simulink model "Demo_CarRealTime2D_cs"  (R2014b)
settings: Solver=ode5  SolverMode=SingleTasking  StartTime=0.0  StopTime=inf  FixedStep=1/1000  RelTol=1e-3
PreLoadFcn:
  | mbxruntime.callbacks.PreLoadFcn(bdroot);
  | check_NUTS_defined;
  | assignin('base',['model_closed_' bdroot],false);
  | addpath('../includes_AEBS');
PostLoadFcn:
  | mbxruntime.callbacks.PostLoadFcn(bdroot);
InitFcn:
  | mbxruntime.callbacks.InitFcn(bdroot);
StartFcn:
  | mbxruntime.callbacks.StartFcn(bdroot);
StopFcn:
  | mbxruntime.callbacks.StopFcn(bdroot);;
  | 
model workspace: external: MAT-File .\Demo_CarRealTime2D_cs_hws.mat (data not in the file)
undefined symbols (not defined in the file or in its folder): Driver_Demands, mbxruntime, tabledata, vicrt_initcallback, vicrt_initmexcallback, vicrt_simulationmanager, warningInitialVelocity, x0
undefined symbols (not defined in the file): Demo_CarRealTime2D_cs_007c1c37f387f47f, Demo_CarRealTime2D_cs_085a64a83ba38cec, Demo_CarRealTime2D_cs_0a7f542d3fc7ab9f, Demo_CarRealTime2D_cs_0d7c72cfaa56dff7, Demo_CarRealTime2D_cs_0de07b35068e3828, Demo_CarRealTime2D_cs_17f4d381375cce95, Demo_CarRealTime2D_cs_1db40a09b08215a9, Demo_CarRealTime2D_cs_2bfa3850c176687b, Demo_CarRealTime2D_cs_35a34f1ba6ce4a22, Demo_CarRealTime2D_cs_378cc77e08d643fb, Demo_CarRealTime2D_cs_409b5c3befba0000, Demo_CarRealTime2D_cs_42628ca5bb62d2f3, Demo_CarRealTime2D_cs_56554a2db408a7f8, Demo_CarRealTime2D_cs_59527455249d7429, Demo_CarRealTime2D_cs_5983ee1b8112afac, Demo_CarRealTime2D_cs_5b5ebcf3ed7bf8e6, Demo_CarRealTime2D_cs_63cbe7fbe16cd5d9, Demo_CarRealTime2D_cs_6e17b9adbf989abf, Demo_CarRealTime2D_cs_6f662a34e5d9a196, Demo_CarRealTime2D_cs_75c4ee8892821e19, Demo_CarRealTime2D_cs_7c64486355814be2, Demo_CarRealTime2D_cs_849809550a2230ef, Demo_CarRealTime2D_cs_87f899bcbe16d8f5, Demo_CarRealTime2D_cs_8e7b50dac25b68a2, Demo_CarRealTime2D_cs_94938e5260f139b3, Demo_CarRealTime2D_cs_983acc940698d1d1, Demo_CarRealTime2D_cs_9d554c72797f76fd, Demo_CarRealTime2D_cs_9d747ee2f15c057f, Demo_CarRealTime2D_cs_ad62a2084d31e898, Demo_CarRealTime2D_cs_b56c8c5f000d30f0, Demo_CarRealTime2D_cs_b95f1b7356e926cc, Demo_CarRealTime2D_cs_BMW_X5_1_Path_pathUniqueID, Demo_CarRealTime2D_cs_BMW_Z3_2_Dynamics_Empty_STATE_BMW_Z3_2_x0, Demo_CarRealTime2D_cs_BMW_Z3_2_Dynamics_Empty_STATE_BMW_Z3_2_y0, Demo_CarRealTime2D_cs_BMW_Z3_2_Dynamics_Empty_STATE_BMW_Z3_2_z0, Demo_CarRealTime2D_cs_BMW_Z3_Path_pathUniqueID, Demo_CarRealTime2D_cs_BMW_Z3_SpeedProfile_speedProfileUniqueID, Demo_CarRealTime2D_cs_c8847ab2e5633224, Demo_CarRealTime2D_cs_c9a0d701286b93fb, Demo_CarRealTime2D_cs_ce758cae7dd1b283, Demo_CarRealTime2D_cs_CrossingPedestrian_Path_pathUniqueID, Demo_CarRealTime2D_cs_CuttingInVehicle_Path_pathUniqueID, Demo_CarRealTime2D_cs_d901ab1c1d2e40bc, Demo_CarRealTime2D_cs_dff70430e5a00a86, Demo_CarRealTime2D_cs_ef038a4f619ad32e, Demo_CarRealTime2D_cs_Female_OverweightAni_1_Path_pathUniqueID, Demo_CarRealTime2D_cs_Ford_Fiesta_1_Path_pathUniqueID, Demo_CarRealTime2D_cs_Ford_FocusWagon_Path_pathUniqueID, Demo_CarRealTime2D_cs_Sphere_1_Dynamics_Empty_STATE_Sphere_1_x0, Demo_CarRealTime2D_cs_Sphere_1_Dynamics_Empty_STATE_Sphere_1_y0, Demo_CarRealTime2D_cs_Sphere_1_Dynamics_Empty_STATE_Sphere_1_z0, WheelL0, WheelL1, WheelR0, WheelR1
libraries: PreScanSimulinkLibrary x15, simulink x15, simulink_extras x15, PreScanUsefulBlocks x2, dspsigops x1
(part 14 of 17)

== system Demo_CarRealTime2D_cs/HostVehicle/Dynamics_UserSpecified/VI-CarRealTime/Input_Bus/Bus2Map ==
  Bus In : Inport
  Bus Selector : BusSelector  OutputSignals=Driver_Demands.str_swa,Subsystem_Activation.Internal_Steering_Column_Activity,Driver_Demands.rack_displacement,Driver_Demands.throttle,Driver_Demands.gear,Driver_Demands.clutch,Driver_Demands.brake,Brake_System_General.brk_mast_cyl_pres,Brake_System_General.brk_bias_front,Driver_Demands.user_maneuver_ID,Driver_Demands.user_input_steering,Driver_Demands.user_input_throttle,Driver_Demands.user_input_braking,Driver_Demands.user_input_gear,Driver_Demands.user_input_clutch,Friction.tire_mu.L1,Friction.tire_mu.L2,Friction.tire_mu.R1,Friction.tire_mu.R2,Subsystem_Activation.Internal_Brake_System_Activity.L1,Brake_System.brk_mmag_sign.L1,Brake_System.brk_mmag_unsign.L1,Brake_System.brk_pres.L1,Brake_System.brk_pres_gain.L1,Brake_System.brk_mu.L1,Subsystem_Activation.Internal_Brake_System_Activity.L2,Brake_System.brk_mmag_sign.L2,Brake_System.brk_mmag_unsign.L2,Brake_System.brk_pres.L2,Brake_System.brk_pres_gain.L2,Brake_System.brk_mu.L2,Subsystem_Activation.Internal_Brake_System_Activity.R1,Brake_System.brk_mmag_sign.R1,Brake_System.brk_mmag_unsign.R1,Brake_System.brk_pres.R1,Brake_System.brk_pres_gain.R1,Brake_System.brk_mu.R1,Subsystem_Activation.Internal_Brake_System_Activity.R2,Brake_System.brk_mmag_sign.R2,Brake_System.brk_mmag_unsign.R2,Brake_System.brk_pres.R2,Brake_System.brk_pres_gain.R2,Brake_System.brk_mu.R2,Hook.Fx.rear,Hook.Fy.rear,Hook.Fz.rear,Hook.Mx.rear,Hook.My.rear,Hook.Mz.rear,Rear_Steering_Actuator_disp.str_swa.left,Rear_Steering_Actuator_disp.str_swa.right,Steering.steer_at_spindle.L1,Steering.steer_at_spindle.L2,Steering.steer_at_spindle.R1,Steering.steer_at_spindle.R2,Subsystem_Activation.Internal_Clutch_Activity,Subsystem_Activation.Internal_Engine_Activity,Subsystem_Activation.Internal_Gearbox_Activity,Engine.engine_omega,Engine.engine_max_trq,Engine.engine_min_trq,Engine.engine_trq,Engine.non_termic_engine_trq,GearBox.transmission_ratio,Clutch.clutch_trq,Clutch.clutch_slip_angle,Antiroll_Bar.activity_flag.front,Antiroll_Bar.activity_flag.rear,Antiroll_Bar.force.front,Antiroll_Bar.force.rear,Subsystem_Activation.Internal_Aero_Activity,Aerodynamic.fx_front,Aerodynamic.fy_front,Aerodynamic.fz_front,Aerodynamic.fx_rear,Aerodynamic.fy_rear,Aerodynamic.fz_rear,Aerodynamic.fx_center,Aerodynamic.fy_center,Aerodynamic.fz_center,Aerodynamic.mx,Aerodynamic.my,Aerodynamic.mz,Irregularity.road.L1,Irregularity.road.L2,Irregularity.road.R1,Irregularity.road.R2,Main_Damper.force.L1,Main_Damper.activity_flag.L1,Main_Damper.force.L2,Main_Damper.activity_flag.L2,Main_Damper.force.R1,Main_Damper.activity_flag.R1,Main_Damper.force.R2,Main_Damper.activity_flag.R2,Main_Spring.force.L1,Main_Spring.activity_flag.L1,Main_Spring.force.L2,Main_Spring.activity_flag.L2,Main_Spring.force.R1,Main_Spring.activity_flag.R1,Main_Spring.force.R2,Main_Spring.activity_flag.R2,Main_Bumpstop.force.L1,Main_Bumpstop.activity_flag.L1,Main_Bumpstop.force.L2,Main_Bumpstop.activity_flag.L2,Main_Bumpstop.force.R1,Main_Bumpstop.activity_flag.R1,Main_Bumpstop.force.R2,Main_Bumpstop.activity_flag.R2,Main_Reboundstop.force.L1,Main_Reboundstop.activity_flag.L1,Main_Reboundstop.force.L2,Main_Reboundstop.activity_flag.L2,Main_Reboundstop.force.R1,Main_Reboundstop.activity_flag.R1,Main_Reboundstop.force.R2,Main_Reboundstop.activity_flag.R2,Auxiliary_vertical.force.L1,Auxiliary_vertical.activity_flag.L1,Auxiliary_vertical.force.L2,Auxiliary_vertical.activity_flag.L2,Auxiliary_vertical.force.R1,Auxiliary_vertical.activity_flag.R1,Auxiliary_vertical.force.R2,Auxiliary_vertical.activity_flag.R2,Third_Element.Damper_force.front,Third_Element.Damper_activity_flag.front,Third_Element.Damper_force.rear,Third_Element.Damper_activity_flag.rear,Third_Element.Spring.front,Third_Element.Spring_activity_flag.front,Third_Element.Spring.rear,Third_Element.Spring_activity_flag.rear,Mono_Element.Damper.front,Mono_Element.Damper_activity_flag.front,Mono_Element.Damper.rear,Mono_Element.Damper_activity_flag.rear,Mono_Element.Inerter.front,Mono_Element.Inerter_activity_flag.front,Mono_Element.Inerter.rear,Mono_Element.Inerter_activity_flag.rear,Mono_Element.Spring.front,Mono_Element.Spring_activity_flag.front,Mono_Element.Spring.rear,Mono_Element.Spring_activity_flag.rear,Mono_Element.Bumpstop_Spring.front,Mono_Element.Bumpstop_Spring_activity_flag.front,Mono_Element.Bumpstop_Spring.rear,Mono_Element.Bumpstop_Spring_activity_flag.rear,Mono_Element.Reboundstop_Spring.front,Mono_Element.Reboundstop_Spring_activity_flag.front,Mono_Element.Reboundstop_Spring.rear,Mono_Element.Reboundstop_Spring_activity_flag.rear,Mono_Element.Bumpstop_Damper.front,Mono_Element.Bumpstop_Damper_activity_flag.front,Mono_Element.Bumpstop_Damper.rear,Mono_Element.Bumpstop_Damper_activity_flag.rear,Mono_Element.Reboundstop_Damper.front,Mono_Element.Reboundstop_Damper_activity_flag.front,Mono_Element.Reboundstop_Damper.rear,Mono_Element.Reboundstop_Damper_activity_flag.rear,Subsystem_Activation.Tire_Force_x.L1,Subsystem_Activation.Tire_Force_y.L1,Subsystem_Activation.Tire_Force_z.L1,Subsystem_Activation.Tire_Moment_x.L1,Subsystem_Activation.Tire_Moment_y.L1,Subsystem_Activation.Tire_Moment_z.L1,Tire_Force.Fx.L1,Tire_Force.Fy.L1,Tire_Force.Fz.L1,Tire_Moment.Mx.L1,Tire_Moment.My.L1,Tire_Moment.Mz.L1,Subsystem_Activation.Tire_Force_x.L2,Subsystem_Activation.Tire_Force_y.L2,Subsystem_Activation.Tire_Force_z.L2,Subsystem_Activation.Tire_Moment_x.L2,Subsystem_Activation.Tire_Moment_y.L2,Subsystem_Activation.Tire_Moment_z.L2,Tire_Force.Fx.L2,Tire_Force.Fy.L2,Tire_Force.Fz.L2,Tire_Moment.Mx.L2,Tire_Moment.My.L2,Tire_Moment.Mz.L2,Subsystem_Activation.Tire_Force_x.R1,Subsystem_Activation.Tire_Force_y.R1,Subsystem_Activation.Tire_Force_z.R1,Subsystem_Activation.Tire_Moment_x.R1,Subsystem_Activation.Tire_Moment_y.R1,Subsystem_Activation.Tire_Moment_z.R1,Tire_Force.Fx.R1,Tire_Force.Fy.R1,Tire_Force.Fz.R1,Tire_Moment.Mx.R1,Tire_Moment.My.R1,Tire_Moment.Mz.R1,Subsystem_Activation.Tire_Force_x.R2,Subsystem_Activation.Tire_Force_y.R2,Subsystem_Activation.Tire_Force_z.R2,Subsystem_Activation.Tire_Moment_x.R2,Subsystem_Activation.Tire_Moment_y.R2,Subsystem_Activation.Tire_Moment_z.R2,Tire_Force.Fx.R2,Tire_Force.Fy.R2,Tire_Force.Fz.R2,Tire_Moment.Mx.R2,Tire_Moment.My.R2,Tire_Moment.Mz.R2,Wheel_driving.moment.L1,Wheel_driving.moment.L2,Wheel_driving.moment.R1,Wheel_driving.moment.R2,Ext_Body.force.X,Ext_Body.force.Y,Ext_Body.force.Z,Ext_Body.moment.X,Ext_Body.moment.Y,Ext_Body.moment.Z,Ext_Ground.force.X,Ext_Ground.force.Y,Ext_Ground.force.Z,Ext_Ground.moment.X,Ext_Ground.moment.Y,Ext_Ground.moment.Z,Ext_Tracking.force.X,Ext_Tracking.force.Y,Ext_Tracking.moment.X,Ext_Tracking.moment.Y
  Mux : Mux  Inputs=231
  Map Out : Outport
  wires:
  Bus Selector/231 -> Mux/231  "<Y>"
  Bus Selector/230 -> Mux/230  "<X>"
  Bus Selector/229 -> Mux/229  "<Y>"
  Bus Selector/228 -> Mux/228  "<X>"
  Bus Selector/227 -> Mux/227  "<Z>"
  Bus Selector/226 -> Mux/226  "<Y>"
  Bus Selector/225 -> Mux/225  "<X>"
  Bus Selector/224 -> Mux/224  "<Z>"
  Bus Selector/223 -> Mux/223  "<Y>"
  Bus Selector/222 -> Mux/222  "<X>"
  Bus Selector/221 -> Mux/221  "<Z>"
  Bus Selector/220 -> Mux/220  "<Y>"
  Bus Selector/219 -> Mux/219  "<X>"
  Bus Selector/218 -> Mux/218  "<Z>"
  Bus Selector/217 -> Mux/217  "<Y>"
  Bus Selector/216 -> Mux/216  "<X>"
  Bus Selector/215 -> Mux/215  "<R2>"
  Bus Selector/214 -> Mux/214  "<R1>"
  Bus Selector/213 -> Mux/213  "<L2>"
  Bus Selector/212 -> Mux/212  "<L1>"
  Bus Selector/211 -> Mux/211  "<R2>"
  Bus Selector/210 -> Mux/210  "<R2>"
  Bus Selector/209 -> Mux/209  "<R2>"
  Bus Selector/208 -> Mux/208  "<R2>"
  Bus Selector/207 -> Mux/207  "<R2>"
  Bus Selector/206 -> Mux/206  "<R2>"
  Bus Selector/205 -> Mux/205  "<R2>"
  Bus Selector/204 -> Mux/204  "<R2>"
  Bus Selector/203 -> Mux/203  "<R2>"
  Bus Selector/202 -> Mux/202  "<R2>"
  Bus Selector/201 -> Mux/201  "<R2>"
  Bus Selector/200 -> Mux/200  "<R2>"
  Bus Selector/199 -> Mux/199  "<R1>"
  Bus Selector/198 -> Mux/198  "<R1>"
  Bus Selector/197 -> Mux/197  "<R1>"
  Bus Selector/196 -> Mux/196  "<R1>"
  Bus Selector/195 -> Mux/195  "<R1>"
  Bus Selector/194 -> Mux/194  "<R1>"
  Bus Selector/193 -> Mux/193  "<R1>"
  Bus Selector/192 -> Mux/192  "<R1>"
  Bus Selector/191 -> Mux/191  "<R1>"
  Bus Selector/190 -> Mux/190  "<R1>"
  Bus Selector/189 -> Mux/189  "<R1>"
  Bus Selector/188 -> Mux/188  "<R1>"
  Bus Selector/187 -> Mux/187  "<L2>"
  Bus Selector/186 -> Mux/186  "<L2>"
  Bus Selector/185 -> Mux/185  "<L2>"
  Bus Selector/184 -> Mux/184  "<L2>"
  Bus Selector/183 -> Mux/183  "<L2>"
  Bus Selector/182 -> Mux/182  "<L2>"
  Bus Selector/181 -> Mux/181  "<L2>"
  Bus Selector/180 -> Mux/180  "<L2>"
  Bus Selector/179 -> Mux/179  "<L2>"
  Bus Selector/178 -> Mux/178  "<L2>"
  Bus Selector/177 -> Mux/177  "<L2>"
  Bus Selector/176 -> Mux/176  "<L2>"
  Bus Selector/175 -> Mux/175  "<L1>"
  Bus Selector/174 -> Mux/174  "<L1>"
  Bus Selector/173 -> Mux/173  "<L1>"
  Bus Selector/172 -> Mux/172  "<L1>"
  Bus Selector/171 -> Mux/171  "<L1>"
  Bus Selector/170 -> Mux/170  "<L1>"
  Bus Selector/169 -> Mux/169  "<L1>"
  Bus Selector/168 -> Mux/168  "<L1>"
  Bus Selector/167 -> Mux/167  "<L1>"
  Bus Selector/166 -> Mux/166  "<L1>"
  Bus Selector/165 -> Mux/165  "<L1>"
  Bus Selector/164 -> Mux/164  "<L1>"
  Bus Selector/163 -> Mux/163  "<rear>"
  Bus Selector/162 -> Mux/162  "<rear>"
  Bus Selector/161 -> Mux/161  "<front>"
  Bus Selector/160 -> Mux/160  "<front>"
  Bus Selector/159 -> Mux/159  "<rear>"
  Bus Selector/158 -> Mux/158  "<rear>"
  Bus Selector/157 -> Mux/157  "<front>"
  Bus Selector/156 -> Mux/156  "<front>"
  Bus Selector/155 -> Mux/155  "<rear>"
  Bus Selector/154 -> Mux/154  "<rear>"
  Bus Selector/153 -> Mux/153  "<front>"
  Bus Selector/152 -> Mux/152  "<front>"
  Bus Selector/151 -> Mux/151  "<rear>"
  Bus Selector/150 -> Mux/150  "<rear>"
  Bus Selector/149 -> Mux/149  "<front>"
  Bus Selector/148 -> Mux/148  "<front>"
  Bus Selector/147 -> Mux/147  "<rear>"
  Bus Selector/146 -> Mux/146  "<rear>"
  Bus Selector/145 -> Mux/145  "<front>"
  Bus Selector/144 -> Mux/144  "<front>"
  Bus Selector/143 -> Mux/143  "<rear>"
  Bus Selector/142 -> Mux/142  "<rear>"
  Bus Selector/141 -> Mux/141  "<front>"
  Bus Selector/140 -> Mux/140  "<front>"
  Bus Selector/139 -> Mux/139  "<rear>"
  Bus Selector/138 -> Mux/138  "<rear>"
  Bus Selector/137 -> Mux/137  "<front>"
  Bus Selector/136 -> Mux/136  "<front>"
  Bus Selector/135 -> Mux/135  "<rear>"
  Bus Selector/134 -> Mux/134  "<rear>"
  Bus Selector/133 -> Mux/133  "<front>"
  Bus Selector/132 -> Mux/132  "<front>"
  Bus Selector/131 -> Mux/131  "<rear>"
  Bus Selector/130 -> Mux/130  "<rear>"
  Bus Selector/129 -> Mux/129  "<front>"
  Bus Selector/128 -> Mux/128  "<front>"
  Bus Selector/127 -> Mux/127  "<R2>"
  Bus Selector/126 -> Mux/126  "<R2>"
  Bus Selector/125 -> Mux/125  "<R1>"
  Bus Selector/124 -> Mux/124  "<R1>"
  Bus Selector/123 -> Mux/123  "<L2>"
  Bus Selector/122 -> Mux/122  "<L2>"
  Bus Selector/121 -> Mux/121  "<L1>"
  Bus Selector/120 -> Mux/120  "<L1>"
  Bus Selector/119 -> Mux/119  "<R2>"
  Bus Selector/118 -> Mux/118  "<R2>"
  Bus Selector/117 -> Mux/117  "<R1>"
  Bus Selector/116 -> Mux/116  "<R1>"
  Bus Selector/115 -> Mux/115  "<L2>"
  Bus Selector/114 -> Mux/114  "<L2>"
  Bus Selector/113 -> Mux/113  "<L1>"
  Bus Selector/112 -> Mux/112  "<L1>"
  Bus Selector/111 -> Mux/111  "<R2>"
  Bus Selector/110 -> Mux/110  "<R2>"
  Bus Selector/109 -> Mux/109  "<R1>"
  Bus Selector/108 -> Mux/108  "<R1>"
  Bus Selector/107 -> Mux/107  "<L2>"
  Bus Selector/106 -> Mux/106  "<L2>"
  Bus Selector/105 -> Mux/105  "<L1>"
  Bus Selector/104 -> Mux/104  "<L1>"
  Bus Selector/103 -> Mux/103  "<R2>"
  Bus Selector/102 -> Mux/102  "<R2>"
  Bus Selector/101 -> Mux/101  "<R1>"
  Bus Selector/100 -> Mux/100  "<R1>"
  Bus Selector/99 -> Mux/99  "<L2>"
  Bus Selector/98 -> Mux/98  "<L2>"
  Bus Selector/97 -> Mux/97  "<L1>"
  Bus Selector/96 -> Mux/96  "<L1>"
  Bus Selector/95 -> Mux/95  "<R2>"
  Bus Selector/94 -> Mux/94  "<R2>"
  Bus Selector/93 -> Mux/93  "<R1>"
  Bus Selector/92 -> Mux/92  "<R1>"
  Bus Selector/91 -> Mux/91  "<L2>"
  Bus Selector/90 -> Mux/90  "<L2>"
  Bus Selector/89 -> Mux/89  "<L1>"
  Bus Selector/88 -> Mux/88  "<L1>"
  Bus Selector/87 -> Mux/87  "<R2>"
  Bus Selector/86 -> Mux/86  "<R1>"
  Bus Selector/85 -> Mux/85  "<L2>"
  Bus Selector/84 -> Mux/84  "<L1>"
  Bus Selector/83 -> Mux/83  "<mz>"
  Bus Selector/82 -> Mux/82  "<my>"
  Bus Selector/81 -> Mux/81  "<mx>"
  Bus Selector/80 -> Mux/80  "<fz_center>"
  Bus Selector/79 -> Mux/79  "<fy_center>"
  Bus Selector/78 -> Mux/78  "<fx_center>"
  Bus Selector/77 -> Mux/77  "<fz_rear>"
  Bus Selector/76 -> Mux/76  "<fy_rear>"
  Bus Selector/75 -> Mux/75  "<fx_rear>"
  Bus Selector/74 -> Mux/74  "<fz_front>"
  Bus Selector/73 -> Mux/73  "<fy_front>"
  Bus Selector/72 -> Mux/72  "<fx_front>"
  Bus Selector/71 -> Mux/71  "<Internal_Aero_Activity>"
  Bus Selector/70 -> Mux/70  "<rear>"
  Bus Selector/69 -> Mux/69  "<front>"
  Bus Selector/68 -> Mux/68  "<rear>"
  Bus Selector/67 -> Mux/67  "<front>"
  Bus Selector/66 -> Mux/66  "<clutch_slip_angle>"
  Bus Selector/65 -> Mux/65  "<clutch_trq>"
  Bus Selector/64 -> Mux/64  "<transmission_ratio>"
  Bus Selector/63 -> Mux/63  "<non_termic_engine_trq>"
  Bus Selector/62 -> Mux/62  "<engine_trq>"
  Bus Selector/61 -> Mux/61  "<engine_min_trq>"
  Bus Selector/60 -> Mux/60  "<engine_max_trq>"
  Bus Selector/59 -> Mux/59  "<engine_omega>"
  Bus Selector/58 -> Mux/58  "<Internal_Gearbox_Activity>"
  Bus Selector/57 -> Mux/57  "<Internal_Engine_Activity>"
  Bus Selector/56 -> Mux/56  "<Internal_Clutch_Activity>"
  Bus Selector/55 -> Mux/55  "<R2>"
  Bus Selector/54 -> Mux/54  "<R1>"
  Bus Selector/53 -> Mux/53  "<L2>"
  Bus Selector/52 -> Mux/52  "<L1>"
  Bus Selector/51 -> Mux/51  "<right>"
  Bus Selector/50 -> Mux/50  "<left>"
  Bus Selector/49 -> Mux/49  "<rear>"
  Bus Selector/48 -> Mux/48  "<rear>"
  Bus Selector/47 -> Mux/47  "<rear>"
  Bus Selector/46 -> Mux/46  "<rear>"
  Bus Selector/45 -> Mux/45  "<rear>"
  Bus Selector/44 -> Mux/44  "<rear>"
  Bus Selector/43 -> Mux/43  "<R2>"
  Bus Selector/42 -> Mux/42  "<R2>"
  Bus Selector/41 -> Mux/41  "<R2>"
  Bus Selector/40 -> Mux/40  "<R2>"
  Bus Selector/39 -> Mux/39  "<R2>"
  Bus Selector/38 -> Mux/38  "<R2>"
  Bus Selector/37 -> Mux/37  "<R1>"
  Bus Selector/36 -> Mux/36  "<R1>"
  Bus Selector/35 -> Mux/35  "<R1>"
  Bus Selector/34 -> Mux/34  "<R1>"
  Bus Selector/33 -> Mux/33  "<R1>"
  Bus Selector/32 -> Mux/32  "<R1>"
  Bus Selector/31 -> Mux/31  "<L2>"
  Bus Selector/30 -> Mux/30  "<L2>"
  Bus Selector/29 -> Mux/29  "<L2>"
  Bus Selector/28 -> Mux/28  "<L2>"
  Bus Selector/27 -> Mux/27  "<L2>"
  Bus Selector/26 -> Mux/26  "<L2>"
  Bus Selector/25 -> Mux/25  "<L1>"
  Bus Selector/24 -> Mux/24  "<L1>"
  Bus Selector/23 -> Mux/23  "<L1>"
  Bus Selector/22 -> Mux/22  "<L1>"
  Bus Selector/21 -> Mux/21  "<L1>"
  Bus Selector/20 -> Mux/20  "<L1>"
  Bus Selector/19 -> Mux/19  "<R2>"
  Bus Selector/18 -> Mux/18  "<R1>"
  Bus Selector/17 -> Mux/17  "<L2>"
  Bus Selector/16 -> Mux/16  "<L1>"
  Bus Selector/15 -> Mux/15  "<user_input_clutch>"
  Bus Selector/14 -> Mux/14  "<user_input_gear>"
  Bus Selector/13 -> Mux/13  "<user_input_braking>"
  Bus Selector/12 -> Mux/12  "<user_input_throttle>"
  Bus Selector/11 -> Mux/11  "<user_input_steering>"
  Bus Selector/10 -> Mux/10  "<user_maneuver_ID>"
  Bus Selector/9 -> Mux/9  "<brk_bias_front>"
  Bus Selector/8 -> Mux/8  "<brk_mast_cyl_pres>"
  Bus Selector/7 -> Mux/7  "<brake>"
  Bus Selector/6 -> Mux/6  "<clutch>"
  Bus Selector/5 -> Mux/5  "<gear>"
  Bus Selector/4 -> Mux/4  "<throttle>"
  Bus Selector/3 -> Mux/3  "<rack_displacement>"
  Bus Selector/2 -> Mux/2  "<Internal_Steering_Column_Activity>"
  Bus Selector/1 -> Mux/1  "<str_swa>"
  Bus In/1 -> Bus Selector/1
  Mux/1 -> Map Out/1

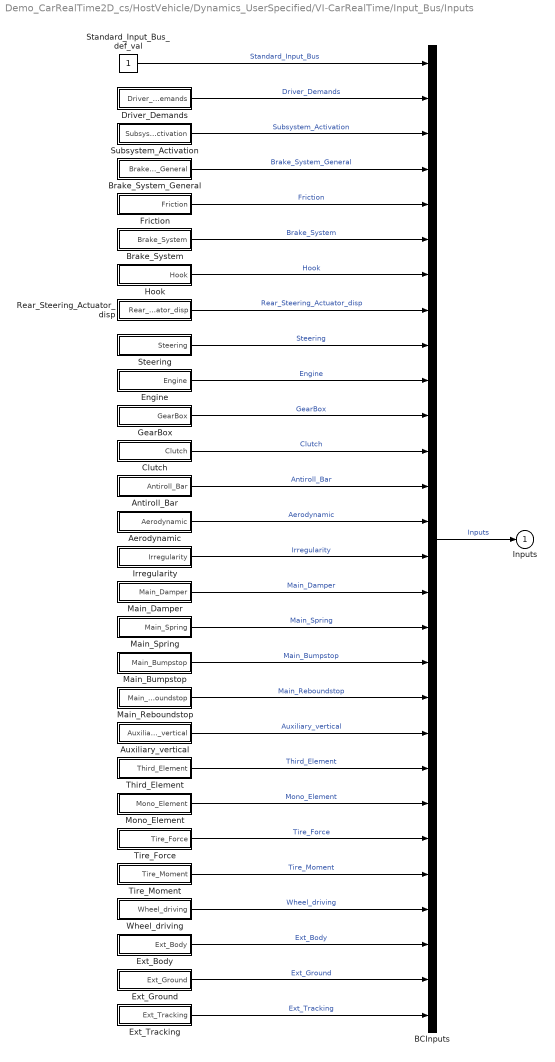
== system Demo_CarRealTime2D_cs/HostVehicle/Dynamics_UserSpecified/VI-CarRealTime/Input_Bus/Inputs ==
  Aerodynamic : Subsystem
  Antiroll_Bar : Subsystem
  Auxiliary_vertical : Subsystem
  BCInputs : BusCreator  Inputs=28
  Brake_System : Subsystem
  Brake_System_General : Subsystem
  Clutch : Subsystem
  Driver_Demands : Subsystem
  Engine : Subsystem
  Ext_Body : Subsystem
  Ext_Ground : Subsystem
  Ext_Tracking : Subsystem
  Friction : Subsystem
  GearBox : Subsystem
  Hook : Subsystem
  Irregularity : Subsystem
  Main_Bumpstop : Subsystem
  Main_Damper : Subsystem
  Main_Reboundstop : Subsystem
  Main_Spring : Subsystem
  Mono_Element : Subsystem
  Rear_Steering_Actuator_disp : Subsystem
  Standard_Input_Bus_def_val : Constant
  Steering : Subsystem
  Subsystem_Activation : Subsystem
  Third_Element : Subsystem
  Tire_Force : Subsystem
  Tire_Moment : Subsystem
  Wheel_driving : Subsystem
  Inputs : Outport
  wires:
  Ext_Tracking/1(Ext_Tracking) -> BCInputs/28  "Ext_Tracking"
  Ext_Ground/1(Ext_Ground) -> BCInputs/27  "Ext_Ground"
  Ext_Body/1(Ext_Body) -> BCInputs/26  "Ext_Body"
  Wheel_driving/1(Wheel_driving) -> BCInputs/25  "Wheel_driving"
  Tire_Moment/1(Tire_Moment) -> BCInputs/24  "Tire_Moment"
  Tire_Force/1(Tire_Force) -> BCInputs/23  "Tire_Force"
  Mono_Element/1(Mono_Element) -> BCInputs/22  "Mono_Element"
  Third_Element/1(Third_Element) -> BCInputs/21  "Third_Element"
  Auxiliary_vertical/1(Auxiliary_vertical) -> BCInputs/20  "Auxiliary_vertical"
  Main_Reboundstop/1(Main_Reboundstop) -> BCInputs/19  "Main_Reboundstop"
  Main_Bumpstop/1(Main_Bumpstop) -> BCInputs/18  "Main_Bumpstop"
  Main_Spring/1(Main_Spring) -> BCInputs/17  "Main_Spring"
  Main_Damper/1(Main_Damper) -> BCInputs/16  "Main_Damper"
  Irregularity/1(Irregularity) -> BCInputs/15  "Irregularity"
  Aerodynamic/1(Aerodynamic) -> BCInputs/14  "Aerodynamic"
  Antiroll_Bar/1(Antiroll_Bar) -> BCInputs/13  "Antiroll_Bar"
  Clutch/1(Clutch) -> BCInputs/12  "Clutch"
  GearBox/1(GearBox) -> BCInputs/11  "GearBox"
  Engine/1(Engine) -> BCInputs/10  "Engine"
  Steering/1(Steering) -> BCInputs/9  "Steering"
  Rear_Steering_Actuator_disp/1(Rear_Steering_Actuator_disp) -> BCInputs/8  "Rear_Steering_Actuator_disp"
  Hook/1(Hook) -> BCInputs/7  "Hook"
  Brake_System/1(Brake_System) -> BCInputs/6  "Brake_System"
  Friction/1(Friction) -> BCInputs/5  "Friction"
  Brake_System_General/1(Brake_System_General) -> BCInputs/4  "Brake_System_General"
  Subsystem_Activation/1(Subsystem_Activation) -> BCInputs/3  "Subsystem_Activation"
  Driver_Demands/1(Driver_Demands) -> BCInputs/2  "Driver_Demands"
  Standard_Input_Bus_def_val/1 -> BCInputs/1  "Standard_Input_Bus"
  BCInputs/1 -> Inputs/1  "Inputs"
